simulink model "Freio_LQR_Model"  (R2025a)
settings: Solver=FixedStepDiscrete  StartTime=0.0  StopTime=3  FixedStep=0.0005  RelTol=1e-3
values from neighbouring files (symbols this model uses):
  Ad = sys_d.A    [ensaio_malha_fechada_lqi.m]
  Bd = sys_d.B    [ensaio_malha_fechada_lqi.m]
  Cd = sys_d.C    [ensaio_malha_fechada_lqi.m]
  Ki = K_aug(3)    [ensaio_malha_fechada_lqi.m]
  Kx = K_aug(1:2)    [ensaio_malha_fechada_lqi.m]
  Ld = place(Ad',Cd',0.4*eig(Ad))'    [ensaio_malha_fechada_lqi.m]
  Pret = 1e5    (= 100000)    [ensaio_integrado_malha_aberta_real.m]    (also in ensaio_malha_fechada_lqi.m)
  Psup_op = Pw_op + 5e5    (= 1500000)    [ensaio_malha_fechada_lqi.m]
  Pw_op = 10e5    (= 1000000)    [ensaio_malha_fechada_lqi.m]
  Ts = Ts_list(i)    [ensaio_malha_fechada_lqi.m]    (also in ensaio_malha_fechada_ruido_medicao.m = evalin('base','Ts'))
undefined symbols (not defined in the file or in its folder): DiscIntNeverNeededParam
libraries: simulink x1
settings Model: Creator=uidq5744  LastModifiedBy=uidq5744

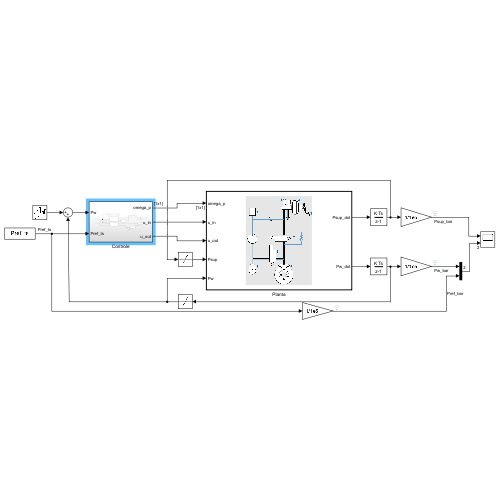
[thumbnail: Simulink's stored preview of the top-level diagram]
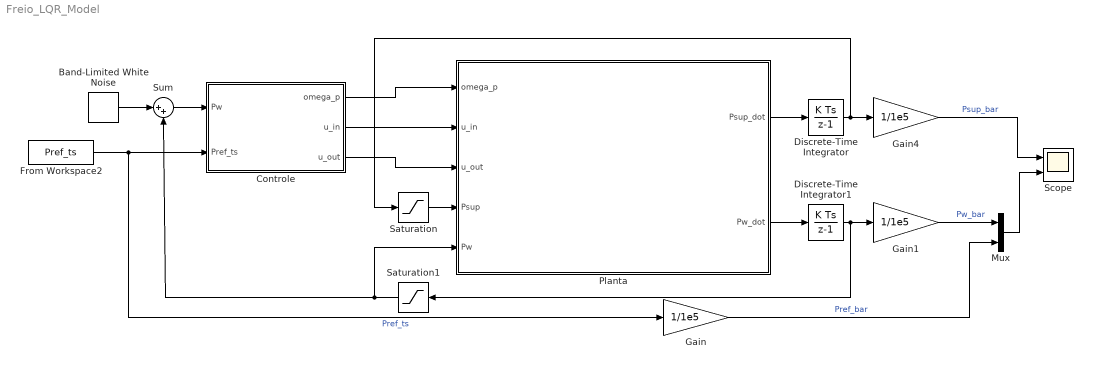
== system Freio_LQR_Model ==
  Band-Limited White Noise : simulink/Sources/Band-Limited White Noise  Cov=5e4  Ts=Ts  seed=[23341]
  Controle : Subsystem
  Discrete-Time Integrator : DiscreteIntegrator  InitialCondition=Psup_op  SampleTime=Ts  ICPrevOutput=DiscIntNeverNeededParam  ICPrevScaledInput=DiscIntNeverNeededParam
  Discrete-Time Integrator1 : DiscreteIntegrator  InitialCondition=Pw_op  SampleTime=Ts  ICPrevOutput=DiscIntNeverNeededParam  ICPrevScaledInput=DiscIntNeverNeededParam
  From Workspace2 : FromWorkspace  VariableName=Pref_ts
  Gain : Gain  Gain=1/1e5
  Gain1 : Gain  Gain=1/1e5
  Gain4 : Gain  Gain=1/1e5
  Mux : Mux  Inputs=2
  Planta : MATLAB Function  TreatAsAtomicUnit=on
  Saturation : Saturate  UpperLimit=Pret + 100e13  LowerLimit=Pret
  Saturation1 : Saturate  UpperLimit=1.5e7  LowerLimit=0
  Scope : Scope  NumInputPorts=2
      settings: ActiveDisplayYMinimum=-11.681391392715879  ActiveDisplayYMaximum=115.13252249693743
  Sum : Sum  Inputs=|++
  wires:
  Planta/1(Psup_dot) -> Discrete-Time Integrator/1
  Planta/2(Pw_dot) -> Discrete-Time Integrator1/1
  Saturation/1 -> Planta/4(Psup)
  Saturation1/1 -> Planta/5(Pw), Sum/2
  Discrete-Time Integrator/1 -> Gain4/1, Saturation/1
  Discrete-Time Integrator1/1 -> Gain1/1, Saturation1/1
  Gain1/1 -> Mux/1  "Pw_bar"
  Gain4/1 -> Scope/1  "Psup_bar"
  From Workspace2/1 -> Gain/1, Controle/2(Pref_ts)  "Pref_ts"
  Gain/1 -> Mux/2  "Pref_bar"
  Mux/1 -> Scope/2
  Band-Limited White Noise/1 -> Sum/1
  Sum/1 -> Controle/1(Pw)
  Controle/1(omega_p) -> Planta/1(omega_p)
  Controle/2(u_in) -> Planta/2(u_in)
  Controle/3(u_out) -> Planta/3(u_out)

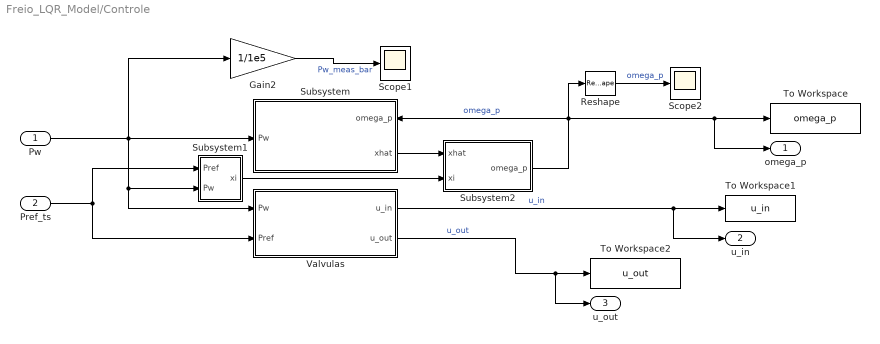
== system Freio_LQR_Model/Controle ==
  Pw : Inport
  Pref_ts : Inport  Port=2
  Gain2 : Gain  Gain=1/1e5
  Reshape : Reshape
  Scope1 : Scope
      settings: ActiveDisplayYMinimum=-11.681391392715879  ActiveDisplayYMaximum=115.13252249693743  DataLoggingVariableName=ScopeData2
  Scope2 : Scope
      settings: ActiveDisplayYMinimum=-187.49999999999997  ActiveDisplayYMaximum=1687.5
  Subsystem : Subsystem
      settings: PortSchema="{\"entries\":[{\"content\":{\"sides\":[{\"content\":{\"connectorIds\":[\"In1\"]},\"type\":\"ConnectorPlacement.EquallySpacedRectSide\",\"uuid\":\"2d02aabb-e49a-4b40-bddc-b8152a05eab8\"},{\"content\":{\"connectorIds\":[\"In2\",\"Out1\"],\"side\":\"RIGHT\"},\"type\":\"ConnectorPlacement.EquallySpacedRectSide\",\"uuid\":\"a50f7af0-a726-4721-9c50-baccf050a1bc\"},{\"content\":{\"side\":\"TOP\"},\"type\":\"ConnectorPlacement.EquallySpacedRectSide\",\"uuid\":\"fa7a67c6-cd9b-48ad-bdd9-afea802f7f75\"}]},\"type\":\"ConnectorPlacement.EquallySpacedConnector\",\"uuid\":\"a18d5477-d2b3-4cd9-a843-769434e14b70\"}],\"packageUris\":[\"http://schema.mathworks.com/mf0/Connector/R2020b\"],\"version\":\"1.0\"}"
  Subsystem1 : Subsystem
  Subsystem2 : Subsystem
  To Workspace : ToWorkspace  VariableName=omega_p  SaveFormat=Timeseries  SampleTime=-1
  To Workspace1 : ToWorkspace  VariableName=u_in  SaveFormat=Timeseries  SampleTime=-1
  To Workspace2 : ToWorkspace  VariableName=u_out  SaveFormat=Timeseries  SampleTime=-1
  Valvulas : MATLAB Function  TreatAsAtomicUnit=on
  omega_p : Outport
  u_in : Outport  Port=2
  u_out : Outport  Port=3
  wires:
  Reshape/1 -> Scope2/1  "omega_p"
  Subsystem2/1(omega_p) -> omega_p/1, To Workspace/1, Subsystem/2(omega_p), Reshape/1  "omega_p"
  Valvulas/2(u_out) -> u_out/1, To Workspace2/1  "u_out"
  Subsystem/1(xhat) -> Subsystem2/1(xhat)
  Pw/1 -> Valvulas/1(Pw), Subsystem1/2(Pw), Subsystem/1(Pw), Gain2/1
  Pref_ts/1 -> Valvulas/2(Pref), Subsystem1/1(Pref)
  Valvulas/1(u_in) -> u_in/1, To Workspace1/1  "u_in"
  Subsystem1/1(xi) -> Subsystem2/2(xi)
  Gain2/1 -> Scope1/1  "Pw_meas_bar"

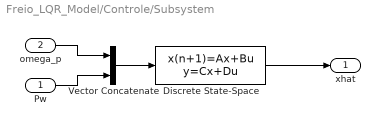
== system Freio_LQR_Model/Controle/Subsystem ==
  Pw : Inport
  omega_p : Inport  Port=2
  Discrete State-Space : DiscreteStateSpace  A=Ad - Ld*Cd  B=[Bd Ld]  C=eye(2)  D=zeros(2,2)  SampleTime=-1
  Vector Concatenate : Concatenate  Mode=Multidimensional array
  xhat : Outport
  wires:
  Pw/1 -> Vector Concatenate/2
  omega_p/1 -> Vector Concatenate/1
  Vector Concatenate/1 -> Discrete State-Space/1
  Discrete State-Space/1 -> xhat/1

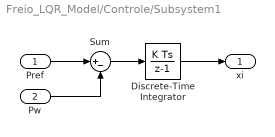
== system Freio_LQR_Model/Controle/Subsystem1 ==
  Pref : Inport
  Pw : Inport  Port=2
  Discrete-Time Integrator : DiscreteIntegrator  SampleTime=Ts  ICPrevOutput=DiscIntNeverNeededParam  ICPrevScaledInput=DiscIntNeverNeededParam
  Sum : Sum  Inputs=|+-
  xi : Outport
  wires:
  Discrete-Time Integrator/1 -> xi/1
  Pw/1 -> Sum/2
  Sum/1 -> Discrete-Time Integrator/1
  Pref/1 -> Sum/1

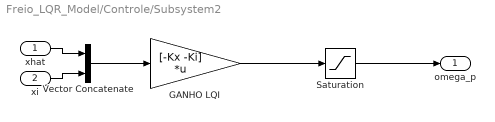
== system Freio_LQR_Model/Controle/Subsystem2 ==
  xhat : Inport
  xi : Inport  Port=2
  GANHO LQI : Gain  Gain=[-Kx -Ki]  Multiplication=Matrix(K*u)
  Saturation : Saturate  UpperLimit=1500  LowerLimit=0
  Vector Concatenate : Concatenate  Mode=Multidimensional array
  omega_p : Outport
  wires:
  xhat/1 -> Vector Concatenate/1
  xi/1 -> Vector Concatenate/2
  Vector Concatenate/1 -> GANHO LQI/1
  Saturation/1 -> omega_p/1
  GANHO LQI/1 -> Saturation/1

== matlab function Freio_LQR_Model/Planta ==
  data: omega_p input; Psup_dot output; u_in input; u_out input; Psup input; Pw input; Pw_dot output
function [Psup_dot, Pw_dot] = Bloco_Hidraulico_2P(omega_p, u_in, u_out, Psup, Pw)
% omega_p: rad/s (>=0)
% u_in, u_out: 0..1 (PWM normalizado / abertura proporcional)
% Psup, Pw: Pa
% Saídas: derivadas de pressão e vazões (m^3/s)

% ---------- parâmetros hidráulicos básicos ----------
beta = 1.5e9;   % Pa - módulo volumétrico efetivo (óleo + mangueiras)
rho  = 850;     % kg/m^3 - densidade típica de fluido de freio
Pret = 1e5;     % Pa - pressão de retorno (aprox. atmosférica)

% ---------- volumes efetivos ----------
% Ordens de grandeza compatíveis com circuitos de freio/HCU:
% - Lv2014, ChenLv2017: pequenas câmaras, respostas de 80–300 MPa/s.
%
% Vsup: volume efetivo do manifold/suprimento (linha de alta + câmara da HCU)
% Vw  : volume efetivo do circuito "roda"/caliper (câmara da pinça + linha)
Vsup = 6.0e-5;   % m^3  (~100 mL)
Vw   = 1.0e-5;   % m^3  (~10 mL)

% ---------- bomba (modelo linear simples) ----------
% Referência: bombas de HCU/IEB com deslocamentos da ordem de 0.1–1 cm^3/volta,
% vazões < 1 L/min em regimes típicos (WangBingbing2015, MotorParametricDesign2023).
%
Dp_rev = 5e-7;           % m^3/rev (0.5 cm^3/1000 rev; pequeno deslocamento por volta)
Nv     = 0.85;           % eficiência volumétrica
Kb     = Nv * (Dp_rev/(2*pi));   % m^3/rad  (Qpump = Kb*omega_p)
Klb    = 1e-11;          % (m^3/s)/Pa - vazamento interno equivalente

% ---------- válvulas (lei do orifício) ----------
% Coerente com diâmetros de ~0.6–0.8 mm (ChenLv2017, ProportionalPressureABS2023):
% A = pi*(d/2)^2. Para d ≈ 0.7 mm -> A ≈ 3.8e-7 m^2.
% Usamos área máxima ligeiramente menor para representar abertura efetiva.
Cv_in   = 0.62;          % coeficiente de descarga típico
Cv_out  = 0.62;
Ain_max = 3.0e-7;        % m^2 - área máx. da válvula de entrada
Aout_max= 3.0e-7;        % m^2 - área máx. da válvula de saída

% Vazamentos opcionais (para estabilidade numérica / perdas pequenas)
Kleak_sup = 1e-15;           % (m^3/s)/Pa
Kleak_w   = 1e-15;           % (m^3/s)/Pa

% ---------- sanitização de entradas ----------
if omega_p < 0
    omega_p = 0;
end
u_in  = min(max(u_in,  0), 1);
u_out = min(max(u_out, 0), 1);

% Evita pressões abaixo do retorno (numérico)
Psup = max(Psup, Pret);
Pw   = max(Pw,   Pret);

% ---------- bomba -> suprimento ----------
Qpump = Kb*omega_p - Klb*(Psup - Pret);
% Nota: usa (Psup - Pret) para não "puxar" abaixo da pressão de retorno.

% ---------- suprimento -> roda (válvula de entrada) ----------
dPin = max(Psup - Pw, 0);
Qin  = Cv_in * (Ain_max * u_in) * sqrt(2*dPin/rho);

% ---------- roda -> retorno (válvula de saída) ----------
dPout = max(Pw - Pret, 0);
Qout  = Cv_out * (Aout_max * u_out) * sqrt(2*dPout/rho);

% ---------- dinâmica das pressões ----------
Psup_dot = (beta/Vsup) * ( Qpump - Qin - Kleak_sup*(Psup - Pret) );
Pw_dot   = (beta/Vw)   * ( Qin - Qout - Kleak_w*(Pw   - Pret) );
end

== matlab function Freio_LQR_Model/Controle/Valvulas ==
  data: Pw input; Pref input; u_in output; u_out output
function [u_in,u_out] = Valvulas(Pw,Pref)

delta_on  = 2e5;
delta_off = 1e5;

persistent state

if isempty(state)
    state = 0;
end

erro = Pref - Pw;

switch state
    
    case 0
        if erro > delta_on
            state = 1;
        elseif erro < -delta_on
            state = -1;
        end
        
    case 1
        if erro < delta_off
            state = 0;
        end
        
    case -1
        if erro > -delta_off
            state = 0;
        end
        
end

u_in  = double(state == 1);
u_out = double(state == -1);

end
